simulink model "Modello_Irb1300_Test"  (R2024a)
settings: Solver=VariableStepAuto  StartTime=0.0  StopTime=30.0  RelTol=1e-3
undefined symbols (not defined in the file or in its folder): DiscIntNeverNeededParam
libraries: simulink x1, vrlib x1
settings Model: Creator=giaki  LastModifiedBy=giaki

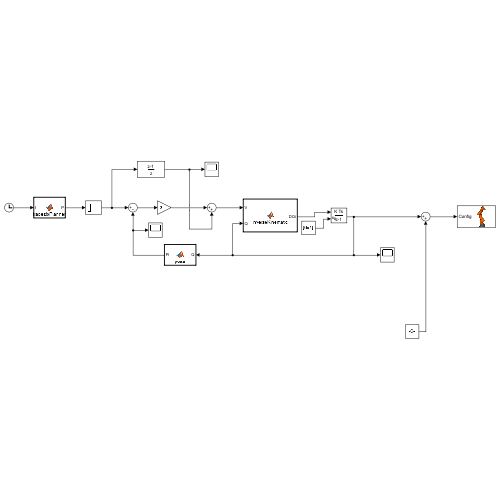
[thumbnail: Simulink's stored preview of the top-level diagram]
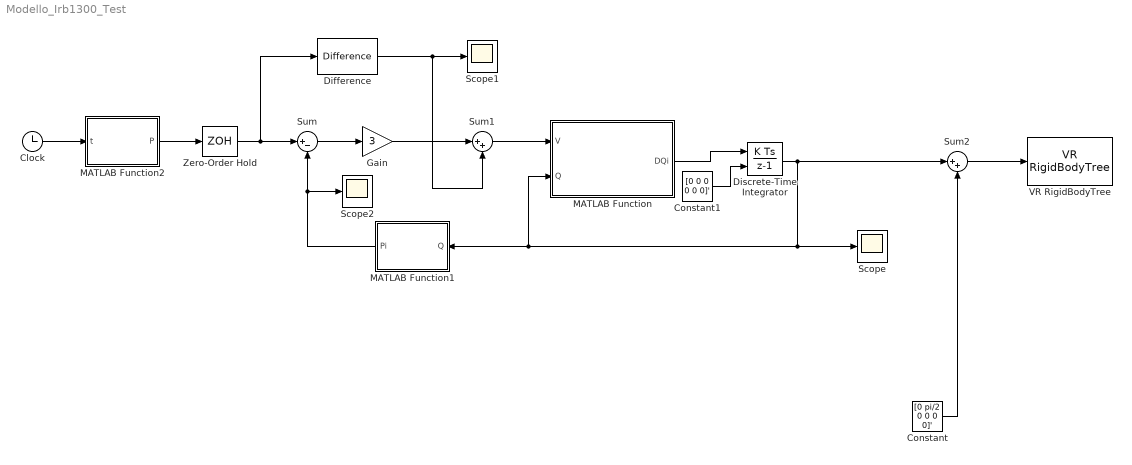
== system Modello_Irb1300_Test ==
  Clock : Clock
  Constant : Constant  Value=[0 pi/2 0 0 0 0]'
  Constant1 : Constant  Value=[0 0 0 0 0 0]'
  Difference : simulink/Discrete/Difference  ICPrevInput=[0.66 0 1.01].'  OutMin=[]  OutMax=[]  OutDataType=fixdt(1, 16)  OutScaling=2^-10  DoSatur=off
  Discrete-Time Integrator : DiscreteIntegrator  InitialConditionSource=external  SampleTime=-1  OutMin=[2]  ICPrevOutput=DiscIntNeverNeededParam  ICPrevScaledInput=DiscIntNeverNeededParam
  Gain : Gain  Gain=3
  MATLAB Function : MATLAB Function  TreatAsAtomicUnit=on
  MATLAB Function1 : MATLAB Function  TreatAsAtomicUnit=on
  MATLAB Function2 : MATLAB Function  TreatAsAtomicUnit=on
  Scope : Scope
  Scope1 : Scope
  Scope2 : Scope
  Sum : Sum  Inputs=|+-
  Sum1 : Sum  Inputs=|++
  Sum2 : Sum  Inputs=|++
  VR RigidBodyTree : vrlib/VR RigidBodyTree  VrmlFile=robot_scene_2.x3d  RBT=Irb1300  useRBT=on  Ts=0.1  ForceViewerOpen=on
  Zero-Order Hold : ZeroOrderHold  SampleTime=0.05
  wires:
  Sum1/1 -> MATLAB Function/1(V)
  Discrete-Time Integrator/1 -> MATLAB Function/2(Q), MATLAB Function1/1(Q), Scope/1, Sum2/1
  Constant/1 -> Sum2/2
  MATLAB Function2/1(P) -> Zero-Order Hold/1
  Constant1/1 -> Discrete-Time Integrator/2
  Difference/1 -> Scope1/1, Sum1/2
  Sum/1 -> Gain/1
  MATLAB Function1/1(Pi) -> Scope2/1, Sum/2
  Zero-Order Hold/1 -> Difference/1, Sum/1
  Clock/1 -> MATLAB Function2/1(t)
  MATLAB Function/1(DQi) -> Discrete-Time Integrator/1
  Gain/1 -> Sum1/1
  Sum2/1 -> VR RigidBodyTree/1

== matlab function Modello_Irb1300_Test/MATLAB Function ==
  data: V input; DQi output; Q input
function DQi = inverseKinematic(V,Q)

th1 = Q(1);
th2 = Q(2);
th3 = Q(3);
th4 = Q(4);
th5 = Q(5);
th6 = Q(6);

% Jacobian evaluated every time in the position Q
% viene chiamato J ma il jacobiano seguente è in verità il jacobiano di
% poszione Jp 
% J = [
% [(9*sin(th5)*(cos(th1)*sin(th4) - cos(th4)*(cos(th3)*cos(th2 + pi/2)*sin(th1) - sin(th1)*sin(th3)*sin(th2 + pi/2))))/100 - (17*cos(th2 + pi/2)*sin(th1))/40 - sin(th1)/20 - (9*cos(th5)*(cos(th3)*sin(th1)*sin(th2 + pi/2) + cos(th2 + pi/2)*sin(th1)*sin(th3)))/100 - (cos(th3)*cos(th2 + pi/2)*sin(th1))/25 - (17*cos(th3)*sin(th1)*sin(th2 + pi/2))/40 - (17*cos(th2 + pi/2)*sin(th1)*sin(th3))/40 + (sin(th1)*sin(th3)*sin(th2 + pi/2))/25, (17*cos(th1)*cos(th3)*cos(th2 + pi/2))/40 - (9*cos(th5)*(cos(th1)*sin(th3)*sin(th2 + pi/2) - cos(th1)*cos(th3)*cos(th2 + pi/2)))/100 - (cos(th1)*cos(th3)*sin(th2 + pi/2))/25 - (cos(th1)*cos(th2 + pi/2)*sin(th3))/25 - (17*cos(th1)*sin(th3)*sin(th2 + pi/2))/40 - (9*cos(th4)*sin(th5)*(cos(th1)*cos(th3)*sin(th2 + pi/2) + cos(th1)*cos(th2 + pi/2)*sin(th3)))/100 - (17*cos(th1)*sin(th2 + pi/2))/40, (17*cos(th1)*cos(th3)*cos(th2 + pi/2))/40 - (cos(th1)*cos(th3)*sin(th2 + pi/2))/25 - (cos(th1)*cos(th2 + pi/2)*sin(th3))/25 - (17*cos(th1)*sin(th3)*sin(th2 + pi/2))/40 - (9*cos(th4)*sin(th5)*(cos(th1)*cos(th3)*sin(th2 + pi/2) + cos(th1)*cos(th2 + pi/2)*sin(th3)))/100 - (9*cos(th5)*(cos(th1)*sin(th3)*sin(th2 + pi/2) - cos(th1)*cos(th3)*cos(th2 + pi/2)))/100,  (9*sin(th5)*(cos(th4)*sin(th1) + sin(th4)*(cos(th1)*sin(th3)*sin(th2 + pi/2) - cos(th1)*cos(th3)*cos(th2 + pi/2))))/100,   (9*cos(th5)*(sin(th1)*sin(th4) - cos(th4)*(cos(th1)*sin(th3)*sin(th2 + pi/2) - cos(th1)*cos(th3)*cos(th2 + pi/2))))/100 - (9*sin(th5)*(cos(th1)*cos(th3)*sin(th2 + pi/2) + cos(th1)*cos(th2 + pi/2)*sin(th3)))/100, 0]
% [cos(th1)/20 + (17*cos(th1)*cos(th2 + pi/2))/40 + (9*sin(th5)*(sin(th1)*sin(th4) - cos(th4)*(cos(th1)*sin(th3)*sin(th2 + pi/2) - cos(th1)*cos(th3)*cos(th2 + pi/2))))/100 + (9*cos(th5)*(cos(th1)*cos(th3)*sin(th2 + pi/2) + cos(th1)*cos(th2 + pi/2)*sin(th3)))/100 + (17*cos(th1)*cos(th3)*sin(th2 + pi/2))/40 + (17*cos(th1)*cos(th2 + pi/2)*sin(th3))/40 - (cos(th1)*sin(th3)*sin(th2 + pi/2))/25 + (cos(th1)*cos(th3)*cos(th2 + pi/2))/25, (9*cos(th5)*(cos(th3)*cos(th2 + pi/2)*sin(th1) - sin(th1)*sin(th3)*sin(th2 + pi/2)))/100 - (17*sin(th1)*sin(th2 + pi/2))/40 + (17*cos(th3)*cos(th2 + pi/2)*sin(th1))/40 - (cos(th3)*sin(th1)*sin(th2 + pi/2))/25 - (cos(th2 + pi/2)*sin(th1)*sin(th3))/25 - (17*sin(th1)*sin(th3)*sin(th2 + pi/2))/40 - (9*cos(th4)*sin(th5)*(cos(th3)*sin(th1)*sin(th2 + pi/2) + cos(th2 + pi/2)*sin(th1)*sin(th3)))/100, (9*cos(th5)*(cos(th3)*cos(th2 + pi/2)*sin(th1) - sin(th1)*sin(th3)*sin(th2 + pi/2)))/100 + (17*cos(th3)*cos(th2 + pi/2)*sin(th1))/40 - (cos(th3)*sin(th1)*sin(th2 + pi/2))/25 - (cos(th2 + pi/2)*sin(th1)*sin(th3))/25 - (17*sin(th1)*sin(th3)*sin(th2 + pi/2))/40 - (9*cos(th4)*sin(th5)*(cos(th3)*sin(th1)*sin(th2 + pi/2) + cos(th2 + pi/2)*sin(th1)*sin(th3)))/100, -(9*sin(th5)*(cos(th1)*cos(th4) + sin(th4)*(cos(th3)*cos(th2 + pi/2)*sin(th1) - sin(th1)*sin(th3)*sin(th2 + pi/2))))/100, - (9*cos(th5)*(cos(th1)*sin(th4) - cos(th4)*(cos(th3)*cos(th2 + pi/2)*sin(th1) - sin(th1)*sin(th3)*sin(th2 + pi/2))))/100 - (9*sin(th5)*(cos(th3)*sin(th1)*sin(th2 + pi/2) + cos(th2 + pi/2)*sin(th1)*sin(th3)))/100, 0]
% [                                                                                                                                                                                                                                                                                                                                                                                                                                            0,                                                                                  (17*cos(th2 + pi/2))/40 + (cos(th3)*cos(th2 + pi/2))/25 + (17*cos(th3)*sin(th2 + pi/2))/40 + (17*cos(th2 + pi/2)*sin(th3))/40 - (sin(th3)*sin(th2 + pi/2))/25 + (9*cos(th5)*(cos(th3)*sin(th2 + pi/2) + cos(th2 + pi/2)*sin(th3)))/100 + (9*cos(th4)*sin(th5)*(cos(th3)*cos(th2 + pi/2) - sin(th3)*sin(th2 + pi/2)))/100,                                                                         (cos(th3)*cos(th2 + pi/2))/25 + (17*cos(th3)*sin(th2 + pi/2))/40 + (17*cos(th2 + pi/2)*sin(th3))/40 - (sin(th3)*sin(th2 + pi/2))/25 + (9*cos(th5)*(cos(th3)*sin(th2 + pi/2) + cos(th2 + pi/2)*sin(th3)))/100 + (9*cos(th4)*sin(th5)*(cos(th3)*cos(th2 + pi/2) - sin(th3)*sin(th2 + pi/2)))/100,                                         -(9*sin(th4)*sin(th5)*(cos(th3)*sin(th2 + pi/2) + cos(th2 + pi/2)*sin(th3)))/100,                                                             (9*sin(th5)*(cos(th3)*cos(th2 + pi/2) - sin(th3)*sin(th2 + pi/2)))/100 + (9*cos(th4)*cos(th5)*(cos(th3)*sin(th2 + pi/2) + cos(th2 + pi/2)*sin(th3)))/100, 0]
% ];
% J = [
% [(9*sin(th5)*(cos(th1)*sin(th4) - cos(th4)*(cos(th3)*cos(th2 + pi/2)*sin(th1) - sin(th1)*sin(th3)*sin(th2 + pi/2))))/100 - (17*cos(th2 + pi/2)*sin(th1))/40 - sin(th1)/20 - (9*cos(th5)*(cos(th3)*sin(th1)*sin(th2 + pi/2) + cos(th2 + pi/2)*sin(th1)*sin(th3)))/100 - (cos(th3)*cos(th2 + pi/2)*sin(th1))/25 - (17*cos(th3)*sin(th1)*sin(th2 + pi/2))/40 - (17*cos(th2 + pi/2)*sin(th1)*sin(th3))/40 + (sin(th1)*sin(th3)*sin(th2 + pi/2))/25, (17*cos(th1)*cos(th3)*cos(th2 + pi/2))/40 - (9*cos(th5)*(cos(th1)*sin(th3)*sin(th2 + pi/2) - cos(th1)*cos(th3)*cos(th2 + pi/2)))/100 - (cos(th1)*cos(th3)*sin(th2 + pi/2))/25 - (cos(th1)*cos(th2 + pi/2)*sin(th3))/25 - (17*cos(th1)*sin(th3)*sin(th2 + pi/2))/40 - (9*cos(th4)*sin(th5)*(cos(th1)*cos(th3)*sin(th2 + pi/2) + cos(th1)*cos(th2 + pi/2)*sin(th3)))/100 - (17*cos(th1)*sin(th2 + pi/2))/40, (17*cos(th1)*cos(th3)*cos(th2 + pi/2))/40 - (cos(th1)*cos(th3)*sin(th2 + pi/2))/25 - (cos(th1)*cos(th2 + pi/2)*sin(th3))/25 - (17*cos(th1)*sin(th3)*sin(th2 + pi/2))/40 - (9*cos(th4)*sin(th5)*(cos(th1)*cos(th3)*sin(th2 + pi/2) + cos(th1)*cos(th2 + pi/2)*sin(th3)))/100 - (9*cos(th5)*(cos(th1)*sin(th3)*sin(th2 + pi/2) - cos(th1)*cos(th3)*cos(th2 + pi/2)))/100,  (9*sin(th5)*(cos(th4)*sin(th1) + sin(th4)*(cos(th1)*sin(th3)*sin(th2 + pi/2) - cos(th1)*cos(th3)*cos(th2 + pi/2))))/100,   (9*cos(th5)*(sin(th1)*sin(th4) - cos(th4)*(cos(th1)*sin(th3)*sin(th2 + pi/2) - cos(th1)*cos(th3)*cos(th2 + pi/2))))/100 - (9*sin(th5)*(cos(th1)*cos(th3)*sin(th2 + pi/2) + cos(th1)*cos(th2 + pi/2)*sin(th3)))/100, 0]
% [cos(th1)/20 + (17*cos(th1)*cos(th2 + pi/2))/40 + (9*sin(th5)*(sin(th1)*sin(th4) - cos(th4)*(cos(th1)*sin(th3)*sin(th2 + pi/2) - cos(th1)*cos(th3)*cos(th2 + pi/2))))/100 + (9*cos(th5)*(cos(th1)*cos(th3)*sin(th2 + pi/2) + cos(th1)*cos(th2 + pi/2)*sin(th3)))/100 + (17*cos(th1)*cos(th3)*sin(th2 + pi/2))/40 + (17*cos(th1)*cos(th2 + pi/2)*sin(th3))/40 - (cos(th1)*sin(th3)*sin(th2 + pi/2))/25 + (cos(th1)*cos(th3)*cos(th2 + pi/2))/25, (9*cos(th5)*(cos(th3)*cos(th2 + pi/2)*sin(th1) - sin(th1)*sin(th3)*sin(th2 + pi/2)))/100 - (17*sin(th1)*sin(th2 + pi/2))/40 + (17*cos(th3)*cos(th2 + pi/2)*sin(th1))/40 - (cos(th3)*sin(th1)*sin(th2 + pi/2))/25 - (cos(th2 + pi/2)*sin(th1)*sin(th3))/25 - (17*sin(th1)*sin(th3)*sin(th2 + pi/2))/40 - (9*cos(th4)*sin(th5)*(cos(th3)*sin(th1)*sin(th2 + pi/2) + cos(th2 + pi/2)*sin(th1)*sin(th3)))/100, (9*cos(th5)*(cos(th3)*cos(th2 + pi/2)*sin(th1) - sin(th1)*sin(th3)*sin(th2 + pi/2)))/100 + (17*cos(th3)*cos(th2 + pi/2)*sin(th1))/40 - (cos(th3)*sin(th1)*sin(th2 + pi/2))/25 - (cos(th2 + pi/2)*sin(th1)*sin(th3))/25 - (17*sin(th1)*sin(th3)*sin(th2 + pi/2))/40 - (9*cos(th4)*sin(th5)*(cos(th3)*sin(th1)*sin(th2 + pi/2) + cos(th2 + pi/2)*sin(th1)*sin(th3)))/100, -(9*sin(th5)*(cos(th1)*cos(th4) + sin(th4)*(cos(th3)*cos(th2 + pi/2)*sin(th1) - sin(th1)*sin(th3)*sin(th2 + pi/2))))/100, - (9*cos(th5)*(cos(th1)*sin(th4) - cos(th4)*(cos(th3)*cos(th2 + pi/2)*sin(th1) - sin(th1)*sin(th3)*sin(th2 + pi/2))))/100 - (9*sin(th5)*(cos(th3)*sin(th1)*sin(th2 + pi/2) + cos(th2 + pi/2)*sin(th1)*sin(th3)))/100, 0]
% [                                                                                                                                                                                                                                                                                                                                                                                                                                            0,                                                                                  (17*cos(th2 + pi/2))/40 + (cos(th3)*cos(th2 + pi/2))/25 + (17*cos(th3)*sin(th2 + pi/2))/40 + (17*cos(th2 + pi/2)*sin(th3))/40 - (sin(th3)*sin(th2 + pi/2))/25 + (9*cos(th5)*(cos(th3)*sin(th2 + pi/2) + cos(th2 + pi/2)*sin(th3)))/100 + (9*cos(th4)*sin(th5)*(cos(th3)*cos(th2 + pi/2) - sin(th3)*sin(th2 + pi/2)))/100,                                                                         (cos(th3)*cos(th2 + pi/2))/25 + (17*cos(th3)*sin(th2 + pi/2))/40 + (17*cos(th2 + pi/2)*sin(th3))/40 - (sin(th3)*sin(th2 + pi/2))/25 + (9*cos(th5)*(cos(th3)*sin(th2 + pi/2) + cos(th2 + pi/2)*sin(th3)))/100 + (9*cos(th4)*sin(th5)*(cos(th3)*cos(th2 + pi/2) - sin(th3)*sin(th2 + pi/2)))/100,                                         -(9*sin(th4)*sin(th5)*(cos(th3)*sin(th2 + pi/2) + cos(th2 + pi/2)*sin(th3)))/100,                                                             (9*sin(th5)*(cos(th3)*cos(th2 + pi/2) - sin(th3)*sin(th2 + pi/2)))/100 + (9*cos(th4)*cos(th5)*(cos(th3)*sin(th2 + pi/2) + cos(th2 + pi/2)*sin(th3)))/100, 0]
% ]; 



%jacobinao calcolato con la terna posizionata sulla pinza al centro del
%punto di aggancio 
J = [
 
[(9*sin(th5)*(cos(th1)*sin(th4) - cos(th4)*(cos(th3)*cos(th2 + pi/2)*sin(th1) - sin(th1)*sin(th3)*sin(th2 + pi/2))))/50 - (17*cos(th2 + pi/2)*sin(th1))/40 - sin(th1)/20 - (9*cos(th5)*(cos(th3)*sin(th1)*sin(th2 + pi/2) + cos(th2 + pi/2)*sin(th1)*sin(th3)))/50 - (cos(th3)*cos(th2 + pi/2)*sin(th1))/25 - (17*cos(th3)*sin(th1)*sin(th2 + pi/2))/40 - (17*cos(th2 + pi/2)*sin(th1)*sin(th3))/40 + (sin(th1)*sin(th3)*sin(th2 + pi/2))/25, (17*cos(th1)*cos(th3)*cos(th2 + pi/2))/40 - (9*cos(th5)*(cos(th1)*sin(th3)*sin(th2 + pi/2) - cos(th1)*cos(th3)*cos(th2 + pi/2)))/50 - (cos(th1)*cos(th3)*sin(th2 + pi/2))/25 - (cos(th1)*cos(th2 + pi/2)*sin(th3))/25 - (17*cos(th1)*sin(th3)*sin(th2 + pi/2))/40 - (9*cos(th4)*sin(th5)*(cos(th1)*cos(th3)*sin(th2 + pi/2) + cos(th1)*cos(th2 + pi/2)*sin(th3)))/50 - (17*cos(th1)*sin(th2 + pi/2))/40, (17*cos(th1)*cos(th3)*cos(th2 + pi/2))/40 - (cos(th1)*cos(th3)*sin(th2 + pi/2))/25 - (cos(th1)*cos(th2 + pi/2)*sin(th3))/25 - (17*cos(th1)*sin(th3)*sin(th2 + pi/2))/40 - (9*cos(th4)*sin(th5)*(cos(th1)*cos(th3)*sin(th2 + pi/2) + cos(th1)*cos(th2 + pi/2)*sin(th3)))/50 - (9*cos(th5)*(cos(th1)*sin(th3)*sin(th2 + pi/2) - cos(th1)*cos(th3)*cos(th2 + pi/2)))/50,  (9*sin(th5)*(cos(th4)*sin(th1) + sin(th4)*(cos(th1)*sin(th3)*sin(th2 + pi/2) - cos(th1)*cos(th3)*cos(th2 + pi/2))))/50,   (9*cos(th5)*(sin(th1)*sin(th4) - cos(th4)*(cos(th1)*sin(th3)*sin(th2 + pi/2) - cos(th1)*cos(th3)*cos(th2 + pi/2))))/50 - (9*sin(th5)*(cos(th1)*cos(th3)*sin(th2 + pi/2) + cos(th1)*cos(th2 + pi/2)*sin(th3)))/50, 0]
[cos(th1)/20 + (17*cos(th1)*cos(th2 + pi/2))/40 + (9*sin(th5)*(sin(th1)*sin(th4) - cos(th4)*(cos(th1)*sin(th3)*sin(th2 + pi/2) - cos(th1)*cos(th3)*cos(th2 + pi/2))))/50 + (9*cos(th5)*(cos(th1)*cos(th3)*sin(th2 + pi/2) + cos(th1)*cos(th2 + pi/2)*sin(th3)))/50 + (17*cos(th1)*cos(th3)*sin(th2 + pi/2))/40 + (17*cos(th1)*cos(th2 + pi/2)*sin(th3))/40 - (cos(th1)*sin(th3)*sin(th2 + pi/2))/25 + (cos(th1)*cos(th3)*cos(th2 + pi/2))/25, (9*cos(th5)*(cos(th3)*cos(th2 + pi/2)*sin(th1) - sin(th1)*sin(th3)*sin(th2 + pi/2)))/50 - (17*sin(th1)*sin(th2 + pi/2))/40 + (17*cos(th3)*cos(th2 + pi/2)*sin(th1))/40 - (cos(th3)*sin(th1)*sin(th2 + pi/2))/25 - (cos(th2 + pi/2)*sin(th1)*sin(th3))/25 - (17*sin(th1)*sin(th3)*sin(th2 + pi/2))/40 - (9*cos(th4)*sin(th5)*(cos(th3)*sin(th1)*sin(th2 + pi/2) + cos(th2 + pi/2)*sin(th1)*sin(th3)))/50, (9*cos(th5)*(cos(th3)*cos(th2 + pi/2)*sin(th1) - sin(th1)*sin(th3)*sin(th2 + pi/2)))/50 + (17*cos(th3)*cos(th2 + pi/2)*sin(th1))/40 - (cos(th3)*sin(th1)*sin(th2 + pi/2))/25 - (cos(th2 + pi/2)*sin(th1)*sin(th3))/25 - (17*sin(th1)*sin(th3)*sin(th2 + pi/2))/40 - (9*cos(th4)*sin(th5)*(cos(th3)*sin(th1)*sin(th2 + pi/2) + cos(th2 + pi/2)*sin(th1)*sin(th3)))/50, -(9*sin(th5)*(cos(th1)*cos(th4) + sin(th4)*(cos(th3)*cos(th2 + pi/2)*sin(th1) - sin(th1)*sin(th3)*sin(th2 + pi/2))))/50, - (9*cos(th5)*(cos(th1)*sin(th4) - cos(th4)*(cos(th3)*cos(th2 + pi/2)*sin(th1) - sin(th1)*sin(th3)*sin(th2 + pi/2))))/50 - (9*sin(th5)*(cos(th3)*sin(th1)*sin(th2 + pi/2) + cos(th2 + pi/2)*sin(th1)*sin(th3)))/50, 0]
[                                                                                                                                                                                                                                                                                                                                                                                                                                          0,                                                                                  (17*cos(th2 + pi/2))/40 + (cos(th3)*cos(th2 + pi/2))/25 + (17*cos(th3)*sin(th2 + pi/2))/40 + (17*cos(th2 + pi/2)*sin(th3))/40 - (sin(th3)*sin(th2 + pi/2))/25 + (9*cos(th5)*(cos(th3)*sin(th2 + pi/2) + cos(th2 + pi/2)*sin(th3)))/50 + (9*cos(th4)*sin(th5)*(cos(th3)*cos(th2 + pi/2) - sin(th3)*sin(th2 + pi/2)))/50,                                                                         (cos(th3)*cos(th2 + pi/2))/25 + (17*cos(th3)*sin(th2 + pi/2))/40 + (17*cos(th2 + pi/2)*sin(th3))/40 - (sin(th3)*sin(th2 + pi/2))/25 + (9*cos(th5)*(cos(th3)*sin(th2 + pi/2) + cos(th2 + pi/2)*sin(th3)))/50 + (9*cos(th4)*sin(th5)*(cos(th3)*cos(th2 + pi/2) - sin(th3)*sin(th2 + pi/2)))/50,                                         -(9*sin(th4)*sin(th5)*(cos(th3)*sin(th2 + pi/2) + cos(th2 + pi/2)*sin(th3)))/50,                                                             (9*sin(th5)*(cos(th3)*cos(th2 + pi/2) - sin(th3)*sin(th2 + pi/2)))/50 + (9*cos(th4)*cos(th5)*(cos(th3)*sin(th2 + pi/2) + cos(th2 + pi/2)*sin(th3)))/50, 0]
];  



DQi = pinv(J)*V; % Matlab function for thr pseudo-inverse Matrix
pause (0.01);

end

== matlab function Modello_Irb1300_Test/MATLAB Function2 ==
  data: t input; P output
function P = trapezioPlanner(t)

% Intervallo di tempo
ti = 0;
tf = 10;
t = t - ti;  % Trasformazione del tempo
tf = tf - ti;

% Punti in spazio cartesiano
Pi = [0.66 0 1.01].';     % Posizione iniziale 3x1 (m) la stessa posizione nel riferimento dalla scena è Pi = [0.374 0.63 0]'.
Pf = [0.66 0 1.01].'; % Posizione finale 3x1 (m) Pf = [0.374 0 0.63].'       
P_pos = Pi;                % inzializzo P_pos con la posizione iniziale 

% Differenza di posizione
delta_P = Pf - Pi;

% Parametri per l'orientamento (angoli RPY: Roll, Pitch, Yaw)
% phi = 0; % Angolo di roll (attorno all'asse X) 0;
% theta = 1.5; % Angolo di pitch (attorno all'asse Y) 1.5;
% psi = -1.5; % Angolo di yaw (attorno all'asse Z) -1.5;

% Accelerazione (aggiunta un 10% per garantire che l'accelerazione sia maggiore del valore di riferimento)
Acc = (4 * delta_P / (tf^2)) * 1.1;

% Calcolo degli intervalli di rampa per la traiettoria trapezoidale
tc1 = tf / 2 - sqrt(tf^2 / 4 - norm(delta_P) / norm(Acc));
tc2 = tf / 2 + sqrt(tf^2 / 4 - norm(delta_P) / norm(Acc));


% Calcolo della traiettoria in funzione del tempo
if t >= 0 && t < tc1
    P_pos = Pi + 1/2 * Acc * t^2; % Posizione durante la rampa
elseif t >= tc1 && t < tc2
    P_pos = Pi + Acc * tc1 * (t - tc1 / 2); % Posizione in fase di movimento
elseif t >= tc2 && t < tf
    P_pos = Pf - 1/2 * Acc * (tf - t)^2; % Posizione finale
elseif t >= tf
    P_pos = Pf; % Posizione a tempo finale
end
% L'orientamento viene restituito come angoli RPY (Roll, Pitch, Yaw)
%orientation = [phi; theta; psi];  % Angoli RPY (3x1)

% Uscita: combinazione di posizione (3x1) e orientamento (3x1)
%P = [P_pos; orientation];  % Posizione e orientamento come un vettore 6x1
P = P_pos;
end

== matlab function Modello_Irb1300_Test/MATLAB Function1 ==
  data: Q input; Pi output
function Pi = posa(Q)

th1 = Q(1);
th2 = Q(2);
th3 = Q(3);
th4 = Q(4);
th5 = Q(5);
th6 = Q(6);

% matrix 4x4 evaluated in the position Q
% matriceUtilizzata T06 calcolata con la terna posizionata sulla pinza al centro del
%punto di aggancio 

T = [
[  sin(th6)*(cos(th4)*sin(th1) + sin(th4)*(cos(th1)*sin(th3)*sin(th2 + pi/2) - cos(th1)*cos(th3)*cos(th2 + pi/2))) + cos(th6)*(cos(th5)*(sin(th1)*sin(th4) - cos(th4)*(cos(th1)*sin(th3)*sin(th2 + pi/2) - cos(th1)*cos(th3)*cos(th2 + pi/2))) - sin(th5)*(cos(th1)*cos(th3)*sin(th2 + pi/2) + cos(th1)*cos(th2 + pi/2)*sin(th3))), cos(th6)*(cos(th4)*sin(th1) + sin(th4)*(cos(th1)*sin(th3)*sin(th2 + pi/2) - cos(th1)*cos(th3)*cos(th2 + pi/2))) - sin(th6)*(cos(th5)*(sin(th1)*sin(th4) - cos(th4)*(cos(th1)*sin(th3)*sin(th2 + pi/2) - cos(th1)*cos(th3)*cos(th2 + pi/2))) - sin(th5)*(cos(th1)*cos(th3)*sin(th2 + pi/2) + cos(th1)*cos(th2 + pi/2)*sin(th3))), sin(th5)*(sin(th1)*sin(th4) - cos(th4)*(cos(th1)*sin(th3)*sin(th2 + pi/2) - cos(th1)*cos(th3)*cos(th2 + pi/2))) + cos(th5)*(cos(th1)*cos(th3)*sin(th2 + pi/2) + cos(th1)*cos(th2 + pi/2)*sin(th3)), cos(th1)/20 + (17*cos(th1)*cos(th2 + pi/2))/40 + (9*sin(th5)*(sin(th1)*sin(th4) - cos(th4)*(cos(th1)*sin(th3)*sin(th2 + pi/2) - cos(th1)*cos(th3)*cos(th2 + pi/2))))/50 + (9*cos(th5)*(cos(th1)*cos(th3)*sin(th2 + pi/2) + cos(th1)*cos(th2 + pi/2)*sin(th3)))/50 + (17*cos(th1)*cos(th3)*sin(th2 + pi/2))/40 + (17*cos(th1)*cos(th2 + pi/2)*sin(th3))/40 - (cos(th1)*sin(th3)*sin(th2 + pi/2))/25 + (cos(th1)*cos(th3)*cos(th2 + pi/2))/25]
[- sin(th6)*(cos(th1)*cos(th4) + sin(th4)*(cos(th3)*cos(th2 + pi/2)*sin(th1) - sin(th1)*sin(th3)*sin(th2 + pi/2))) - cos(th6)*(cos(th5)*(cos(th1)*sin(th4) - cos(th4)*(cos(th3)*cos(th2 + pi/2)*sin(th1) - sin(th1)*sin(th3)*sin(th2 + pi/2))) + sin(th5)*(cos(th3)*sin(th1)*sin(th2 + pi/2) + cos(th2 + pi/2)*sin(th1)*sin(th3))), sin(th6)*(cos(th5)*(cos(th1)*sin(th4) - cos(th4)*(cos(th3)*cos(th2 + pi/2)*sin(th1) - sin(th1)*sin(th3)*sin(th2 + pi/2))) + sin(th5)*(cos(th3)*sin(th1)*sin(th2 + pi/2) + cos(th2 + pi/2)*sin(th1)*sin(th3))) - cos(th6)*(cos(th1)*cos(th4) + sin(th4)*(cos(th3)*cos(th2 + pi/2)*sin(th1) - sin(th1)*sin(th3)*sin(th2 + pi/2))), cos(th5)*(cos(th3)*sin(th1)*sin(th2 + pi/2) + cos(th2 + pi/2)*sin(th1)*sin(th3)) - sin(th5)*(cos(th1)*sin(th4) - cos(th4)*(cos(th3)*cos(th2 + pi/2)*sin(th1) - sin(th1)*sin(th3)*sin(th2 + pi/2))), sin(th1)/20 + (17*cos(th2 + pi/2)*sin(th1))/40 - (9*sin(th5)*(cos(th1)*sin(th4) - cos(th4)*(cos(th3)*cos(th2 + pi/2)*sin(th1) - sin(th1)*sin(th3)*sin(th2 + pi/2))))/50 + (9*cos(th5)*(cos(th3)*sin(th1)*sin(th2 + pi/2) + cos(th2 + pi/2)*sin(th1)*sin(th3)))/50 + (cos(th3)*cos(th2 + pi/2)*sin(th1))/25 + (17*cos(th3)*sin(th1)*sin(th2 + pi/2))/40 + (17*cos(th2 + pi/2)*sin(th1)*sin(th3))/40 - (sin(th1)*sin(th3)*sin(th2 + pi/2))/25]
[                                                                                                    cos(th6)*(sin(th5)*(cos(th3)*cos(th2 + pi/2) - sin(th3)*sin(th2 + pi/2)) + cos(th4)*cos(th5)*(cos(th3)*sin(th2 + pi/2) + cos(th2 + pi/2)*sin(th3))) - sin(th4)*sin(th6)*(cos(th3)*sin(th2 + pi/2) + cos(th2 + pi/2)*sin(th3)),                                                                                                 - sin(th6)*(sin(th5)*(cos(th3)*cos(th2 + pi/2) - sin(th3)*sin(th2 + pi/2)) + cos(th4)*cos(th5)*(cos(th3)*sin(th2 + pi/2) + cos(th2 + pi/2)*sin(th3))) - cos(th6)*sin(th4)*(cos(th3)*sin(th2 + pi/2) + cos(th2 + pi/2)*sin(th3)),                                                           cos(th4)*sin(th5)*(cos(th3)*sin(th2 + pi/2) + cos(th2 + pi/2)*sin(th3)) - cos(th5)*(cos(th3)*cos(th2 + pi/2) - sin(th3)*sin(th2 + pi/2)),                                                                                                             (17*sin(th2 + pi/2))/40 - (17*cos(th3)*cos(th2 + pi/2))/40 + (cos(th3)*sin(th2 + pi/2))/25 + (cos(th2 + pi/2)*sin(th3))/25 + (17*sin(th3)*sin(th2 + pi/2))/40 - (9*cos(th5)*(cos(th3)*cos(th2 + pi/2) - sin(th3)*sin(th2 + pi/2)))/50 + (9*cos(th4)*sin(th5)*(cos(th3)*sin(th2 + pi/2) + cos(th2 + pi/2)*sin(th3)))/50 + 68/125]
[                                                                                                                                                                                                                                                                                                                                0,                                                                                                                                                                                                                                                                                                                               0,                                                                                                                                                                                                  0,                                                                                                                                                                                                                                                                                                                                                                                                                                           1]
   ];

% T = [
% [  sin(th6)*(cos(th4)*sin(th1) + sin(th4)*(cos(th1)*sin(th3)*sin(th2 + pi/2) - cos(th1)*cos(th3)*cos(th2 + pi/2))) + cos(th6)*(cos(th5)*(sin(th1)*sin(th4) - cos(th4)*(cos(th1)*sin(th3)*sin(th2 + pi/2) - cos(th1)*cos(th3)*cos(th2 + pi/2))) - sin(th5)*(cos(th1)*cos(th3)*sin(th2 + pi/2) + cos(th1)*cos(th2 + pi/2)*sin(th3))), cos(th6)*(cos(th4)*sin(th1) + sin(th4)*(cos(th1)*sin(th3)*sin(th2 + pi/2) - cos(th1)*cos(th3)*cos(th2 + pi/2))) - sin(th6)*(cos(th5)*(sin(th1)*sin(th4) - cos(th4)*(cos(th1)*sin(th3)*sin(th2 + pi/2) - cos(th1)*cos(th3)*cos(th2 + pi/2))) - sin(th5)*(cos(th1)*cos(th3)*sin(th2 + pi/2) + cos(th1)*cos(th2 + pi/2)*sin(th3))), sin(th5)*(sin(th1)*sin(th4) - cos(th4)*(cos(th1)*sin(th3)*sin(th2 + pi/2) - cos(th1)*cos(th3)*cos(th2 + pi/2))) + cos(th5)*(cos(th1)*cos(th3)*sin(th2 + pi/2) + cos(th1)*cos(th2 + pi/2)*sin(th3)), cos(th1)/20 + (17*cos(th1)*cos(th2 + pi/2))/40 + (9*sin(th5)*(sin(th1)*sin(th4) - cos(th4)*(cos(th1)*sin(th3)*sin(th2 + pi/2) - cos(th1)*cos(th3)*cos(th2 + pi/2))))/100 + (9*cos(th5)*(cos(th1)*cos(th3)*sin(th2 + pi/2) + cos(th1)*cos(th2 + pi/2)*sin(th3)))/100 + (17*cos(th1)*cos(th3)*sin(th2 + pi/2))/40 + (17*cos(th1)*cos(th2 + pi/2)*sin(th3))/40 - (cos(th1)*sin(th3)*sin(th2 + pi/2))/25 + (cos(th1)*cos(th3)*cos(th2 + pi/2))/25]
% [- sin(th6)*(cos(th1)*cos(th4) + sin(th4)*(cos(th3)*cos(th2 + pi/2)*sin(th1) - sin(th1)*sin(th3)*sin(th2 + pi/2))) - cos(th6)*(cos(th5)*(cos(th1)*sin(th4) - cos(th4)*(cos(th3)*cos(th2 + pi/2)*sin(th1) - sin(th1)*sin(th3)*sin(th2 + pi/2))) + sin(th5)*(cos(th3)*sin(th1)*sin(th2 + pi/2) + cos(th2 + pi/2)*sin(th1)*sin(th3))), sin(th6)*(cos(th5)*(cos(th1)*sin(th4) - cos(th4)*(cos(th3)*cos(th2 + pi/2)*sin(th1) - sin(th1)*sin(th3)*sin(th2 + pi/2))) + sin(th5)*(cos(th3)*sin(th1)*sin(th2 + pi/2) + cos(th2 + pi/2)*sin(th1)*sin(th3))) - cos(th6)*(cos(th1)*cos(th4) + sin(th4)*(cos(th3)*cos(th2 + pi/2)*sin(th1) - sin(th1)*sin(th3)*sin(th2 + pi/2))), cos(th5)*(cos(th3)*sin(th1)*sin(th2 + pi/2) + cos(th2 + pi/2)*sin(th1)*sin(th3)) - sin(th5)*(cos(th1)*sin(th4) - cos(th4)*(cos(th3)*cos(th2 + pi/2)*sin(th1) - sin(th1)*sin(th3)*sin(th2 + pi/2))), sin(th1)/20 + (17*cos(th2 + pi/2)*sin(th1))/40 - (9*sin(th5)*(cos(th1)*sin(th4) - cos(th4)*(cos(th3)*cos(th2 + pi/2)*sin(th1) - sin(th1)*sin(th3)*sin(th2 + pi/2))))/100 + (9*cos(th5)*(cos(th3)*sin(th1)*sin(th2 + pi/2) + cos(th2 + pi/2)*sin(th1)*sin(th3)))/100 + (cos(th3)*cos(th2 + pi/2)*sin(th1))/25 + (17*cos(th3)*sin(th1)*sin(th2 + pi/2))/40 + (17*cos(th2 + pi/2)*sin(th1)*sin(th3))/40 - (sin(th1)*sin(th3)*sin(th2 + pi/2))/25]
% [                                                                                                    cos(th6)*(sin(th5)*(cos(th3)*cos(th2 + pi/2) - sin(th3)*sin(th2 + pi/2)) + cos(th4)*cos(th5)*(cos(th3)*sin(th2 + pi/2) + cos(th2 + pi/2)*sin(th3))) - sin(th4)*sin(th6)*(cos(th3)*sin(th2 + pi/2) + cos(th2 + pi/2)*sin(th3)),                                                                                                 - sin(th6)*(sin(th5)*(cos(th3)*cos(th2 + pi/2) - sin(th3)*sin(th2 + pi/2)) + cos(th4)*cos(th5)*(cos(th3)*sin(th2 + pi/2) + cos(th2 + pi/2)*sin(th3))) - cos(th6)*sin(th4)*(cos(th3)*sin(th2 + pi/2) + cos(th2 + pi/2)*sin(th3)),                                                           cos(th4)*sin(th5)*(cos(th3)*sin(th2 + pi/2) + cos(th2 + pi/2)*sin(th3)) - cos(th5)*(cos(th3)*cos(th2 + pi/2) - sin(th3)*sin(th2 + pi/2)),                                                                                                             (17*sin(th2 + pi/2))/40 - (17*cos(th3)*cos(th2 + pi/2))/40 + (cos(th3)*sin(th2 + pi/2))/25 + (cos(th2 + pi/2)*sin(th3))/25 + (17*sin(th3)*sin(th2 + pi/2))/40 - (9*cos(th5)*(cos(th3)*cos(th2 + pi/2) - sin(th3)*sin(th2 + pi/2)))/100 + (9*cos(th4)*sin(th5)*(cos(th3)*sin(th2 + pi/2) + cos(th2 + pi/2)*sin(th3)))/100 + 68/125]
% [                                                                                                                                                                                                                                                                                                                                0,                                                                                                                                                                                                                                                                                                                               0,                                                                                                                                                                                                  0,                                                                                                                                                                                                                                                                                                                                                                                                                                             1]
% ];



Pi = T(1:3,4);

end
